simulink model "grafica_practica1_ejer1"  (R2021a)
settings: Solver=VariableStepAuto  StartTime=0.0  StopTime=10.0  RelTol=1e-3
settings Model: Creator=andrea  LastModifiedBy=andrea

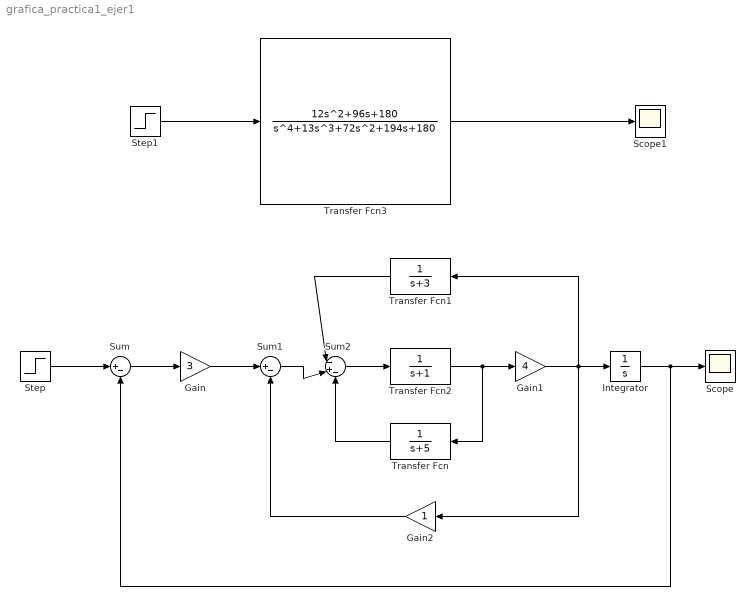
== system grafica_practica1_ejer1 ==
  Gain : Gain  Gain=3
  Gain1 : Gain  Gain=4
  Gain2 : Gain
  Integrator : Integrator
  Scope : Scope
  Scope1 : Scope
  Step : Step  SampleTime=0
  Step1 : Step  SampleTime=0
  Sum : Sum  Inputs=|+-
  Sum1 : Sum  Inputs=|+-
  Sum2 : Sum  Inputs=|-+-
  Transfer Fcn : TransferFcn  Denominator=[1 5]
  Transfer Fcn1 : TransferFcn  Denominator=[1 3]
  Transfer Fcn2 : TransferFcn  Denominator=[1 1]
  Transfer Fcn3 : TransferFcn  Numerator=[12 96 180]  Denominator=[1 13 72 194 180]
  wires:
  Sum2/1 -> Transfer Fcn2/1
  Gain1/1 -> Gain2/1, Transfer Fcn1/1, Integrator/1
  Transfer Fcn2/1 -> Transfer Fcn/1, Gain1/1
  Transfer Fcn/1 -> Sum2/3
  Transfer Fcn1/1 -> Sum2/1
  Gain2/1 -> Sum1/2
  Gain/1 -> Sum1/1
  Sum1/1 -> Sum2/2
  Sum/1 -> Gain/1
  Integrator/1 -> Sum/2, Scope/1
  Step/1 -> Sum/1
  Step1/1 -> Transfer Fcn3/1
  Transfer Fcn3/1 -> Scope1/1
